simulink model "contr3_aprox"  (Simulink 8.5)
settings: Solver=ode3  StartTime=0.0  StopTime=7  FixedStep=0.001  RelTol=1e-3
values from neighbouring files (symbols this model uses):
  K = (y_real(end) - y_real(1))/(input.signals.values(end) - 0)    [ctr.m]
  L = 1.5*(t1_28 - (t2_63/3))    [ctr.m]
  T = 1.5*(t2_63 - t1_28)    [ctr.m]
settings Model: Creator=guima  LastModifiedBy=guima
settings OptimizationCC: ExpressionDepthLimit=128  InitFltsAndDblsToZero=on
settings DebuggingCC: SaveWithParameterizedLinksMsg=none  SignalResolutionControl=TryResolveAllWithWarning  SolverPrmCheckMsg=warning  MultiTaskDSMMsg=warning  MultiTaskCondExecSysMsg=none  FcnCallInpInsideContextMsg=UseLocalSettings  StateNameClashWarn=none  StrictBusMsg=Warning
settings GRTTargetCC: TargetFcnLib=ansi_tfl_tmw.mat

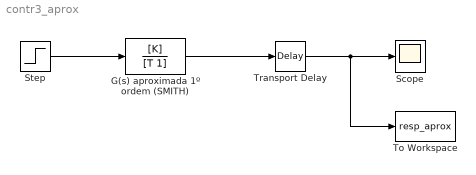
== system contr3_aprox ==
  G(s) aproximada 1º ordem (SMITH) : TransferFcn  Numerator=[K]  Denominator=[T 1]
  Scope : Scope
      settings: MaxDataPoints=7001
  Step : Step  Time=0  SampleTime=0
  To Workspace : ToWorkspace  VariableName=resp_aprox  SaveFormat=Structure With Time  SampleTime=-1
  Transport Delay : TransportDelay  DelayTime=L
  wires:
  Step/1 -> G(s) aproximada 1º ordem (SMITH)/1
  G(s) aproximada 1º ordem (SMITH)/1 -> Transport Delay/1
  Transport Delay/1 -> Scope/1, To Workspace/1
